simulink model "MyMOAB"  (R2021a)
settings: Solver=ode23t  StartTime=0.0  StopTime=Inf  RelTol=1e-3  AbsTol=1e-3
values from neighbouring files (symbols this model uses):
  ball_mass = DEFAULT_BALL_MASS    (= 0.0027)    [MOAB_PARAMS.m]
  ball_moi = calcMOI(ball_radius,ball_shell,ball_mass)    [MOAB_PARAMS.m]
  ball_radius = DEFAULT_BALL_RADIUS    (= 0.02)    [MOAB_PARAMS.m]
  ball_shell = DEFAULT_BALL_SHELL    (= 0.0002)    [MOAB_PARAMS.m]
  DEFAULT_BALL_NOISE = 0.0005    [MOAB_PARAMS.m]
  DEFAULT_GRAVITY = 9.81    [MOAB_PARAMS.m]
  DEFAULT_PLATE_NOISE = 0.0    (= 0)    [MOAB_PARAMS.m]
  DEFAULT_SIMULATION_RATE = 0.2    [MOAB_PARAMS.m]
  DEFAULT_VEL_NOISE = 0.0001    [MOAB_PARAMS.m]
  MAX_ITER = Inf    (= inf)    [MOAB_PARAMS.m]
  noise_mean = 0    [MOAB_PARAMS.m]
  noise_variance = 0.333    [MOAB_PARAMS.m]
  obstacle_radius = DEFAULT_OBSTACLE_RADIUS    (= 0)    [MOAB_PARAMS.m]
  plate_pos_z0 = DEFAULT_PLATE_HEIGHT    (= 0.02)    [MOAB_PARAMS.m]
  plate_radius = DEFAULT_PLATE_RADIUS    (= 0.1125)    [MOAB_PARAMS.m]
  s = 0.1732    [MOAB_PARAMS.m]
  target_pos_x = 0    [MOAB_PARAMS.m]
  target_pos_y = 0    [MOAB_PARAMS.m]
  tilt_acc = DEFAULT_PLATE_ANGULAR_ACCEL    [MOAB_PARAMS.m]
  tilt_limit = DEFAULT_PLATE_ANGLE_LIMIT    [MOAB_PARAMS.m]
  tilt_max_vel = DEFAULT_PLATE_MAX_ANGULAR_VELOCITY    [MOAB_PARAMS.m]
  tilt_x0 = deg2rad(0)    [MOAB_PARAMS.m]
  tilt_y0 = deg2rad(0)    [MOAB_PARAMS.m]
  TIME_DELTA = DEFAULT_SIMULATION_RATE    (= 0.2)    [MOAB_PARAMS.m]
  z_offset = 0.0328538    [MOAB_PARAMS.m]
undefined symbols (not defined in the file or in its folder): smiData, X, Y, Z
libraries: sm_lib x119, nesl_utility x21, simulink x1
(part 4 of 4)

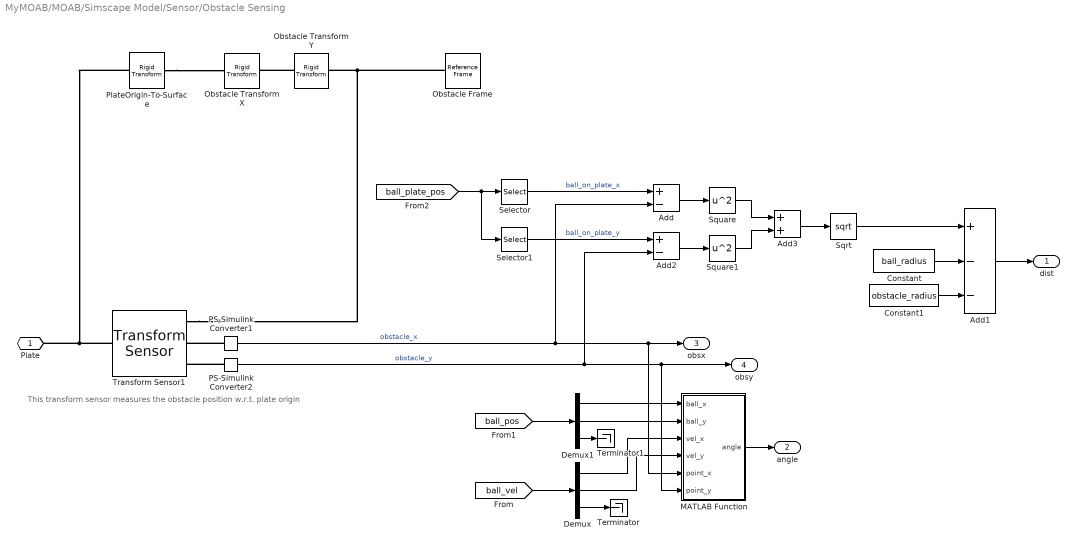
== system MyMOAB/MOAB/Simscape Model/Sensor/Obstacle Sensing ==
  note: This transform sensor measures the obstacle position w.r.t. plate origin
  Add : Sum  Inputs=+-
  Add1 : Sum  Inputs=+--
  Add2 : Sum  Inputs=+-
  Add3 : Sum
  Constant : Constant  Value=ball_radius
  Constant1 : Constant  Value=obstacle_radius
  Demux : Demux  Outputs=3
  Demux1 : Demux  Outputs=3
  MATLAB Function : MATLAB Function  TreatAsAtomicUnit=on
  Obstacle Transform X : sm_lib/Frames and Transforms/Rigid Transform  TranslationMethod=StandardAxis  TranslationStandardOffset=obstacle_pos_x0  TranslationLengthUnit=m  TranslationStandardAxis=+X  TranslationCartesianOffset=[0 0 0]  TranslationROffset=0  TranslationROffsetUnits=m  TranslationZOffset=0  TranslationZOffsetUnits=m  TranslationThetaOffset=0  TranslationThetaOffsetUnits=deg  RotationMethod=None  RotationAngleUnits=deg  RotationStandardAxis=+Z  RotationAngle=0.0  RotationArbitraryAxis=[0 0 1]  FollAlignAxisA=+X  BaseAlignAxisA=+Y  FollAlignAxisB=+Y  BaseAlignAxisB=+Z  RotationSequenceAxes=FollowerAxes  RotationSequence=XYX  RotationSequenceAngles=[0 0 0]  RotationSequenceAnglesUnits=deg  RotationMatrix=[1 0 0; 0 1 0; 0 0 1]
  Obstacle Transform Y : sm_lib/Frames and Transforms/Rigid Transform  TranslationMethod=StandardAxis  TranslationStandardOffset=obstacle_pos_y0  TranslationLengthUnit=m  TranslationStandardAxis=+Y  TranslationCartesianOffset=[0 0 0]  TranslationROffset=0  TranslationROffsetUnits=m  TranslationZOffset=0  TranslationZOffsetUnits=m  TranslationThetaOffset=0  TranslationThetaOffsetUnits=deg  RotationMethod=None  RotationAngleUnits=deg  RotationStandardAxis=+Z  RotationAngle=0.0  RotationArbitraryAxis=[0 0 1]  FollAlignAxisA=+X  BaseAlignAxisA=+Y  FollAlignAxisB=+Y  BaseAlignAxisB=+Z  RotationSequenceAxes=FollowerAxes  RotationSequence=XYX  RotationSequenceAngles=[0 0 0]  RotationSequenceAnglesUnits=deg  RotationMatrix=[1 0 0; 0 1 0; 0 0 1]
  Obstacle Frame : sm_lib/Frames and Transforms/Reference Frame
  PS-Simulink Converter1 : nesl_utility/PS-Simulink Converter  PhysicalDomain=network_engine_domain  SubClassName=ps_output  LeftPortType=input  RightPortType=output  PseudoPeriodic=off  Frequencies=[]  Unit=m  AffineConversion=off
      settings: SourceProductBaseCode=PW,SS
  PS-Simulink Converter2 : nesl_utility/PS-Simulink Converter  PhysicalDomain=network_engine_domain  SubClassName=ps_output  LeftPortType=input  RightPortType=output  PseudoPeriodic=off  Frequencies=[]  Unit=m  AffineConversion=off
      settings: SourceProductBaseCode=PW,SS
  PlateOrigin-To-Surface : sm_lib/Frames and Transforms/Rigid Transform  TranslationMethod=StandardAxis  TranslationStandardOffset=PLATE_ORIGIN_TO_SURFACE_OFFSET  TranslationLengthUnit=m  TranslationStandardAxis=+Z  TranslationCartesianOffset=[0 0 0]  TranslationROffset=0  TranslationROffsetUnits=m  TranslationZOffset=0  TranslationZOffsetUnits=m  TranslationThetaOffset=0  TranslationThetaOffsetUnits=deg  RotationMethod=None  RotationAngleUnits=deg  RotationStandardAxis=+Z  RotationAngle=0.0  RotationArbitraryAxis=[0 0 1]  FollAlignAxisA=+X  BaseAlignAxisA=+Y  FollAlignAxisB=+Y  BaseAlignAxisB=+Z  RotationSequenceAxes=FollowerAxes  RotationSequence=XYX  RotationSequenceAngles=[0 0 0]  RotationSequenceAnglesUnits=deg  RotationMatrix=[1 0 0; 0 1 0; 0 0 1]
  Selector : Selector  InputPortWidth=3  IndexOptions=Index vector (dialog)  Indices=1  OutputSizes=1
  Selector1 : Selector  InputPortWidth=3  IndexOptions=Index vector (dialog)  Indices=2  OutputSizes=1
  Sqrt : Sqrt  SaturateOnIntegerOverflow=on
  Square : Math  Operator=square  SaturateOnIntegerOverflow=on
  Square1 : Math  Operator=square  SaturateOnIntegerOverflow=on
  Terminator : Terminator
  Terminator1 : Terminator
  Transform Sensor1 : sm_lib/Frames and Transforms/Transform Sensor  MeasurementFrame=Base  SenseAngle=off  SenseAxis=off  SenseAngle1=off  SenseAngle2=off  SenseAngle3=off  SenseQ=off  SenseR=off  SenseOmegaX=off  SenseOmegaY=off  SenseOmegaZ=off  SenseOmega1=off  SenseOmega2=off  SenseOmega3=off  SenseQDot=off  SenseRDot=off  SenseAlphaX=off  SenseAlphaY=off  SenseAlphaZ=off  SenseAlpha1=off  SenseAlpha2=off  SenseAlpha3=off  SenseQDDot=off  SenseRDDot=off  SenseX=on  SenseY=on  SenseZ=off  SenseRad=off  SenseAzim=off  SenseDist=off  SenseInc=off  SenseXDot=off  SenseYDot=off  SenseZDot=off  SenseRadDot=off  SenseAzimDot=off  SenseDistDot=off  SenseIncDot=off  SenseXDDot=off  SenseYDDot=off  SenseZDDot=off  SenseRadDDot=off  SenseAzimDDot=off  SenseDistDDot=off  SenseIncDDot=off
  Plate : PMIOPort  Side=Left
  dist : Outport
  angle : Outport  Port=2
  obsx : Outport  Port=3
  obsy : Outport  Port=4
  wires:
  Constant/1 -> Add1/2
  Constant1/1 -> Add1/3
  Add1/1 -> dist/1
  [ball_vel] -> Demux/1
  Demux/2 -> MATLAB Function/4(vel_y)
  Demux/3 -> Terminator/1
  [ball_pos] -> Demux1/1
  Demux1/1 -> MATLAB Function/1(ball_x)
  Demux1/2 -> MATLAB Function/2(ball_y)
  Demux1/3 -> Terminator1/1
  Demux/1 -> MATLAB Function/3(vel_x)
  PS-Simulink Converter1/1 -> obsx/1, MATLAB Function/5(point_x), Add/2  "obstacle_x"
  PS-Simulink Converter2/1 -> MATLAB Function/6(point_y), obsy/1, Add2/2  "obstacle_y"
  MATLAB Function/1(angle) -> angle/1
  [ball_plate_pos] -> Selector1/1, Selector/1
  Selector/1 -> Add/1  "ball_on_plate_x"
  Selector1/1 -> Add2/1  "ball_on_plate_y"
  Add/1 -> Square/1
  Add2/1 -> Square1/1
  Square/1 -> Add3/1
  Square1/1 -> Add3/2
  Add3/1 -> Sqrt/1
  Sqrt/1 -> Add1/1
  connections:
  Obstacle Transform Y/LConn1 -- Obstacle Transform X/RConn1
  Transform Sensor1/LConn1 -- PlateOrigin-To-Surface/LConn1 -- Plate/RConn1
  Obstacle Frame/RConn1 -- Obstacle Transform Y/RConn1 -- Transform Sensor1/RConn1
  PS-Simulink Converter1/LConn1 -- Transform Sensor1/RConn2
  PS-Simulink Converter2/LConn1 -- Transform Sensor1/RConn3
  PlateOrigin-To-Surface/RConn1 -- Obstacle Transform X/LConn1

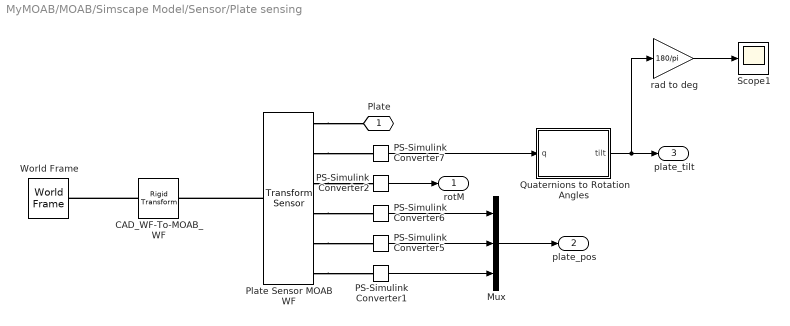
== system MyMOAB/MOAB/Simscape Model/Sensor/Plate sensing ==
  CAD_WF-To-MOAB_WF : sm_lib/Frames and Transforms/Rigid Transform  TranslationMethod=StandardAxis  TranslationStandardOffset=z_offset  TranslationLengthUnit=m  TranslationStandardAxis=+Z  TranslationCartesianOffset=[0 0 0]  TranslationROffset=0  TranslationROffsetUnits=m  TranslationZOffset=0  TranslationZOffsetUnits=m  TranslationThetaOffset=0  TranslationThetaOffsetUnits=deg  RotationMethod=None  RotationAngleUnits=deg  RotationStandardAxis=+Z  RotationAngle=0.0  RotationArbitraryAxis=[0 0 1]  FollAlignAxisA=+X  BaseAlignAxisA=+Y  FollAlignAxisB=+Y  BaseAlignAxisB=+Z  RotationSequenceAxes=FollowerAxes  RotationSequence=XYX  RotationSequenceAngles=[0 0 0]  RotationSequenceAnglesUnits=deg  RotationMatrix=[1 0 0; 0 1 0; 0 0 1]
  Mux : Mux  Inputs=3
  PS-Simulink Converter1 : nesl_utility/PS-Simulink Converter  PhysicalDomain=network_engine_domain  SubClassName=ps_output  LeftPortType=input  RightPortType=output  PseudoPeriodic=off  Frequencies=[]  Unit=m  AffineConversion=off
      settings: SourceProductBaseCode=PW,SS
  PS-Simulink Converter2 : nesl_utility/PS-Simulink Converter  PhysicalDomain=network_engine_domain  SubClassName=ps_output  LeftPortType=input  RightPortType=output  PseudoPeriodic=off  Frequencies=[]  Unit=inherit  AffineConversion=off
      settings: SourceProductBaseCode=PW,SS
  PS-Simulink Converter5 : nesl_utility/PS-Simulink Converter  PhysicalDomain=network_engine_domain  SubClassName=ps_output  LeftPortType=input  RightPortType=output  PseudoPeriodic=off  Frequencies=[]  Unit=m  AffineConversion=off
      settings: SourceProductBaseCode=PW,SS
  PS-Simulink Converter6 : nesl_utility/PS-Simulink Converter  PhysicalDomain=network_engine_domain  SubClassName=ps_output  LeftPortType=input  RightPortType=output  PseudoPeriodic=off  Frequencies=[]  Unit=m  AffineConversion=off
      settings: SourceProductBaseCode=PW,SS
  PS-Simulink Converter7 : nesl_utility/PS-Simulink Converter  PhysicalDomain=network_engine_domain  SubClassName=ps_output  LeftPortType=input  RightPortType=output  PseudoPeriodic=off  Frequencies=[]  Unit=inherit  AffineConversion=off
      settings: SourceProductBaseCode=PW,SS
  Plate Sensor MOAB WF : sm_lib/Frames and Transforms/Transform Sensor  MeasurementFrame=World  SenseAngle=off  SenseAxis=off  SenseAngle1=off  SenseAngle2=off  SenseAngle3=off  SenseQ=on  SenseR=on  SenseOmegaX=off  SenseOmegaY=off  SenseOmegaZ=off  SenseOmega1=off  SenseOmega2=off  SenseOmega3=off  SenseQDot=off  SenseRDot=off  SenseAlphaX=off  SenseAlphaY=off  SenseAlphaZ=off  SenseAlpha1=off  SenseAlpha2=off  SenseAlpha3=off  SenseQDDot=off  SenseRDDot=off  SenseX=on  SenseY=on  SenseZ=on  SenseRad=off  SenseAzim=off  SenseDist=off  SenseInc=off  SenseXDot=off  SenseYDot=off  SenseZDot=off  SenseRadDot=off  SenseAzimDot=off  SenseDistDot=off  SenseIncDot=off  SenseXDDot=off  SenseYDDot=off  SenseZDDot=off  SenseRadDDot=off  SenseAzimDDot=off  SenseDistDDot=off  SenseIncDDot=off
  Quaternions to Rotation Angles : MATLAB Function  TreatAsAtomicUnit=on
  Scope1 : Scope
  World Frame : sm_lib/Frames and Transforms/World Frame
  rad to deg : Gain  Gain=180/pi
  Plate : PMIOPort  Side=Left
  rotM : Outport
  plate_pos : Outport  Port=2
  plate_tilt : Outport  Port=3
  wires:
  PS-Simulink Converter2/1 -> rotM/1
  PS-Simulink Converter7/1 -> Quaternions to Rotation Angles/1(q)
  PS-Simulink Converter5/1 -> Mux/2
  Mux/1 -> plate_pos/1
  PS-Simulink Converter6/1 -> Mux/1
  PS-Simulink Converter1/1 -> Mux/3
  Quaternions to Rotation Angles/1(tilt) -> plate_tilt/1, rad to deg/1
  rad to deg/1 -> Scope1/1
  connections:
  Plate Sensor MOAB WF/RConn6 -- PS-Simulink Converter1/LConn1
  Plate Sensor MOAB WF/RConn5 -- PS-Simulink Converter5/LConn1
  Plate Sensor MOAB WF/RConn1 -- Plate/RConn1
  Plate Sensor MOAB WF/RConn2 -- PS-Simulink Converter7/LConn1
  Plate Sensor MOAB WF/RConn4 -- PS-Simulink Converter6/LConn1
  Plate Sensor MOAB WF/LConn1 -- CAD_WF-To-MOAB_WF/RConn1
  CAD_WF-To-MOAB_WF/LConn1 -- World Frame/RConn1
  Plate Sensor MOAB WF/RConn3 -- PS-Simulink Converter2/LConn1

== matlab function MyMOAB/MOAB/Inverse Kinematics/MATLAB Function ==
  data: plate_height input; alpha output; tilt_x input; tilt_y input; plate_noise input
function alpha = actionsToServoAngles(plate_height, tilt_x, tilt_y, plate_noise)

% add plate noise to x and y tilt
tilt_x = tilt_x + plate_noise;
tilt_y = tilt_y + plate_noise;

% calculate servo joint angles (deg)
[a1,a2,a3] = runMixer(plate_height, tilt_x, tilt_y);

alpha = [a1 a2 a3]';

== matlab function MyMOAB/MOAB/Simscape Model/Sensor/Plate sensing/Quaternions to Rotation Angles ==
  data: q input; tilt output
function tilt = quat2tilt(q)
% Quaternion to Euler angle transformation
% Source: https://en.wikipedia.org/wiki/Conversion_between_quaternions_and_Euler_angles

% unpack quaternion
q0 = q(1);
q1 = q(2);
q2 = q(3);
q3 = q(4);

tilt = zeros(3,1);

% tilt about X axis (tilt_y or roll)
tilt(1) = atan2(2*(q0*q1+q2*q3),1-2*(q1^2+q2^2));

% tilt about Y axis (tilt_x or pitch)
tilt(2) = asin(2*(q0*q2-q3*q1));

% tilt about Z axis (yaw)
tilt(3) = atan2(2*(q0*q3+q2*q1),1-2*(q2^2+q3^2));

== matlab function MyMOAB/MOAB/Simscape Model/Sensor/Obstacle Sensing/MATLAB Function ==
  data: ball_x input; angle output; ball_y input; vel_x input; vel_y input; point_x input; point_y input
function angle = fcn(ball_x, ball_y, vel_x, vel_y, point_x, point_y)

% vector to point
dx = point_x - ball_x;
dy = point_y - ball_y;

% vectors and lengths
u = [dx, dy, 0.0]./norm([dx, dy, 0.0]);
v = [vel_x, vel_y, 0.0]./norm([vel_x, vel_y, 0.0]);
ul = length(u);
vl = length(v);

% no velocity? already on the target?
angle = 0.0;
if (ul ~= 0.0) && (vl ~= 0.0)
    % angle between vectors
    uv_dot = dot(u,v);

    % signed angle
    x = u(1);
    y = u(2);
    angle = atan2(dot([-y, x, 0.0], v), uv_dot);
    if isnan(angle)
        angle = 0.0;
    end
end

== matlab function MyMOAB/MOAB/Direct Kinematics/MATLAB Function ==
  data: alpha input; tilt output; h input
function tilt = alpha2tilt(alpha,h)

s = 0.5 * 0.2 * sqrt(3);    % m, side length of equilateral traingle (calculated from CAD drawing)
L = 0.055;                  % m, arm length of links

zc1 = sin(alpha(1))*2*L;
zc2 = sin(alpha(2))*2*L;
zc3 = sin(alpha(3))*2*L;

R = (zc2+zc3)/2;
tx = asin((zc1-h)*sqrt(3)/s);
ty = asin((zc2-R)*2/s);

tilt = [tx ty];
